simulink model "work2"  (R2020b)
settings: Solver=VariableStepAuto  StartTime=0.0  StopTime=10.0  RelTol=1e-3
settings Model: Creator=99003178  LastModifiedBy=99003178

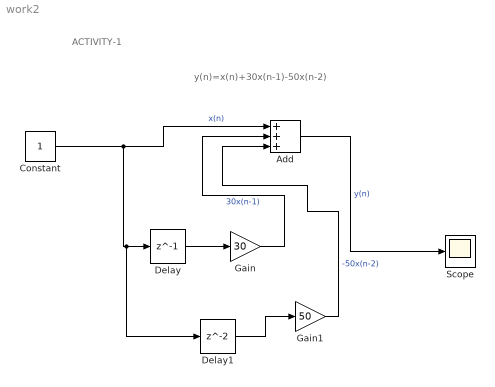
== system work2 ==
  note: y(n)=x(n)+30x(n-1)-50x(n-2)
  note: ACTIVITY-1
  Add : Sum  Inputs=+++
  Constant : Constant
  Delay : Delay  DelayLength=1
  Delay1 : Delay
  Gain : Gain  Gain=30
  Gain1 : Gain  Gain=50
  Scope : Scope
  wires:
  Constant/1 -> Delay1/1, Delay/1, Add/1  "x(n)"
  Add/1 -> Scope/1  "y(n)"
  Delay/1 -> Gain/1
  Delay1/1 -> Gain1/1
  Gain/1 -> Add/2  "30x(n-1)"
  Gain1/1 -> Add/3  "-50x(n-2)"
